simulink model "thuthapdulieu"  (Simulink 9.0)
settings: Solver=FixedStepAuto  StartTime=0.0  StopTime=10000  FixedStep=0.1  RelTol=1e-3
values from neighbouring files (symbols this model uses):
  Kd = 0.1    [thongsohethong.m]
  Ki = 0.01    [thongsohethong.m]
  Kp = 5    [thongsohethong.m]
undefined symbols (not defined in the file or in its folder): DiscIntNeverNeededParam
libraries: simulink x1
settings Model: Creator=TDNhon  LastModifiedBy=DELL
settings DataIOCC: SaveFormat=Dataset  ReturnWorkspaceOutputs=on
settings OptimizationCC: LifeSpan=auto
settings DebuggingCC: UnderspecifiedInitializationDetection=Simplified  MergeDetectMultiDrivingBlocksExec=error  SFUnexpectedBacktrackingDiag=error  SFNoUnconditionalDefaultTransitionDiag=error  SFExecutionAtInitializationDiag=warning
settings HardwareCC: ProdBitPerPointer=64  ProdBitPerSizeT=64  ProdBitPerPtrDiffT=64  ProdLargestAtomicFloat=Float  ProdIntDivRoundTo=Zero  ProdEndianess=LittleEndian  ProdWordSize=64  ProdHWDeviceType=Intel->x86-64 (Windows64)
settings ModelReferenceCC: PropagateSignalLabelsOutOfModel=on
settings SFSimCC: SimUseLocalCustomCode=on
settings RTWCC: RTWUseLocalCustomCode=on
settings CodeAppCC: StateflowObjectComments=off
settings GRTTargetCC: TargetLangStandard=C99 (ISO)
settings ConfigComp: CovMetricSettings=dwe  CovHtmlReporting=off  CovSaveCumulativeToWorkspaceVar=off  CovSaveSingleToWorkspaceVar=off  CovExternalEMLEnable=on

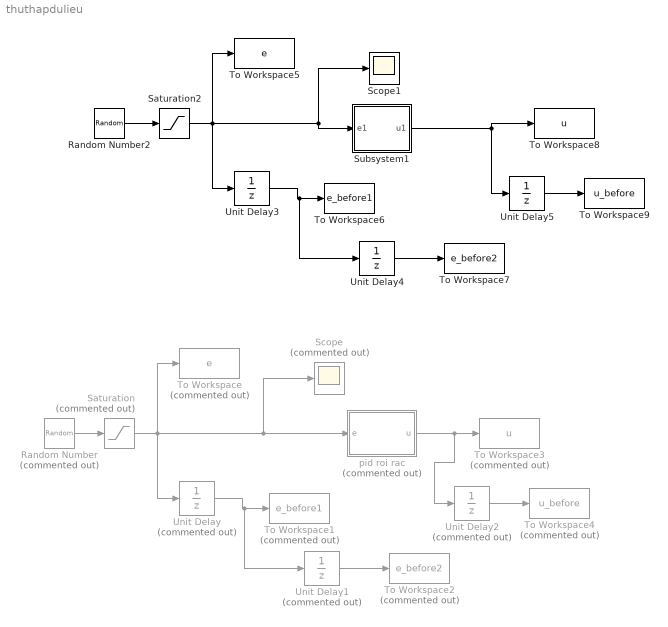
== system thuthapdulieu ==
  Random Number : RandomNumber  Commented=on  Variance=600  Seed=99  SampleTime=0.1
  Random Number2 : RandomNumber  Variance=200  SampleTime=0.1
  Saturation : Saturate  Commented=on  UpperLimit=50  LowerLimit=-50
  Saturation2 : Saturate  UpperLimit=pi/2+0.1  LowerLimit=-pi/2-0.1
  Scope : Scope  Commented=on
  Scope1 : Scope
  Subsystem1 : Subsystem
  To Workspace : ToWorkspace  Commented=on  VariableName=e  SampleTime=-1
  To Workspace1 : ToWorkspace  Commented=on  VariableName=e_before1  SampleTime=-1
  To Workspace2 : ToWorkspace  Commented=on  VariableName=e_before2  SampleTime=-1
  To Workspace3 : ToWorkspace  Commented=on  VariableName=u  SampleTime=-1
  To Workspace4 : ToWorkspace  Commented=on  VariableName=u_before  SampleTime=-1
  To Workspace5 : ToWorkspace  VariableName=e  SampleTime=-1
  To Workspace6 : ToWorkspace  VariableName=e_before1  SampleTime=-1
  To Workspace7 : ToWorkspace  VariableName=e_before2  SampleTime=-1
  To Workspace8 : ToWorkspace  VariableName=u  SampleTime=-1
  To Workspace9 : ToWorkspace  VariableName=u_before  SampleTime=-1
  Unit Delay : UnitDelay  Commented=on  SampleTime=-1
  Unit Delay1 : UnitDelay  Commented=on  SampleTime=-1
  Unit Delay2 : UnitDelay  Commented=on  SampleTime=-1
  Unit Delay3 : UnitDelay  SampleTime=-1
  Unit Delay4 : UnitDelay  SampleTime=-1
  Unit Delay5 : UnitDelay  SampleTime=-1
  pid roi rac : Subsystem  Commented=on
  wires:
  Random Number/1 -> Saturation/1
  Unit Delay/1 -> Unit Delay1/1, To Workspace1/1
  Unit Delay1/1 -> To Workspace2/1
  pid roi rac/1("u ") -> Unit Delay2/1, To Workspace3/1
  Unit Delay2/1 -> To Workspace4/1
  Saturation/1 -> To Workspace/1, Unit Delay/1, Scope/1, pid roi rac/1(e)
  Random Number2/1 -> Saturation2/1
  Unit Delay3/1 -> Unit Delay4/1, To Workspace6/1
  Saturation2/1 -> To Workspace5/1, Unit Delay3/1, Subsystem1/1(e1), Scope1/1
  Subsystem1/1(u1) -> Unit Delay5/1, To Workspace8/1
  Unit Delay5/1 -> To Workspace9/1
  Unit Delay4/1 -> To Workspace7/1

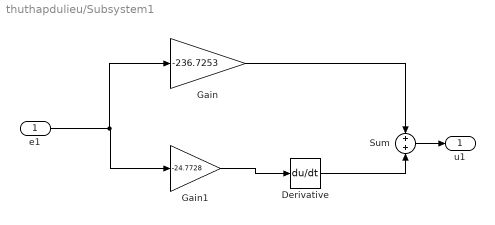
== system thuthapdulieu/Subsystem1 ==
  e1 : Inport
  Derivative : Derivative
  Gain : Gain  Gain=-236.7253
  Gain1 : Gain  Gain=-24.7728
  Sum : Sum
  u1 : Outport
  wires:
  Gain1/1 -> Derivative/1
  e1/1 -> Gain/1, Gain1/1
  Gain/1 -> Sum/1
  Derivative/1 -> Sum/2
  Sum/1 -> u1/1

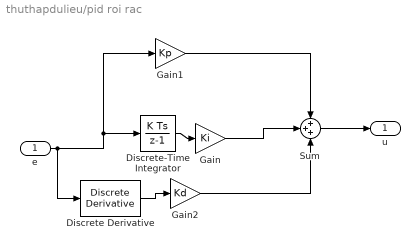
== system thuthapdulieu/pid roi rac ==
  e : Inport
  Discrete Derivative : simulink/Discrete/Discrete Derivative  gainval=1.0  ICPrevScaledInput=0.0  OutMin=[]  OutMax=[]  OutDataType=fixdt(1, 16)  OutScaling=2^-10  DoSatur=off
  Discrete-Time Integrator : DiscreteIntegrator  SampleTime=-1  ICPrevOutput=DiscIntNeverNeededParam  ICPrevScaledInput=DiscIntNeverNeededParam
  Gain : Gain  Gain=Ki
  Gain1 : Gain  Gain=Kp
  Gain2 : Gain  Gain=Kd
  Sum : Sum  Inputs=+++
  "u " : Outport
  wires:
  e/1 -> Discrete Derivative/1, Discrete-Time Integrator/1, Gain1/1
  Discrete-Time Integrator/1 -> Gain/1
  Discrete Derivative/1 -> Gain2/1
  Gain1/1 -> Sum/1
  Gain/1 -> Sum/2
  Gain2/1 -> Sum/3
  Sum/1 -> "u "/1
